simulink model "System23a"  (R2023a)
settings: Solver=ode23t  StartTime=0.0  StopTime=100  MaxStep=0.005  RelTol=1e-3
settings Model: Creator=andriyanov_ilya  LastModifiedBy=Ilya_Andriyanov

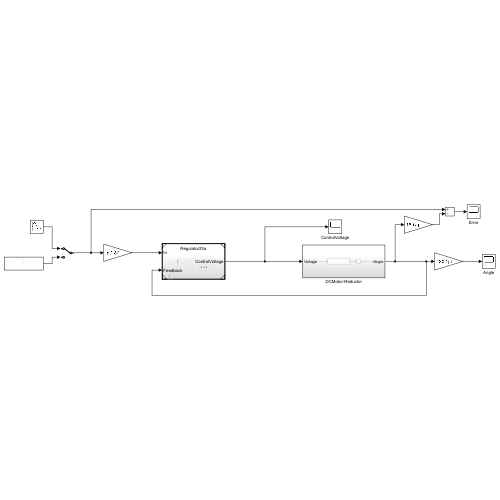
[thumbnail: Simulink's stored preview of the top-level diagram]
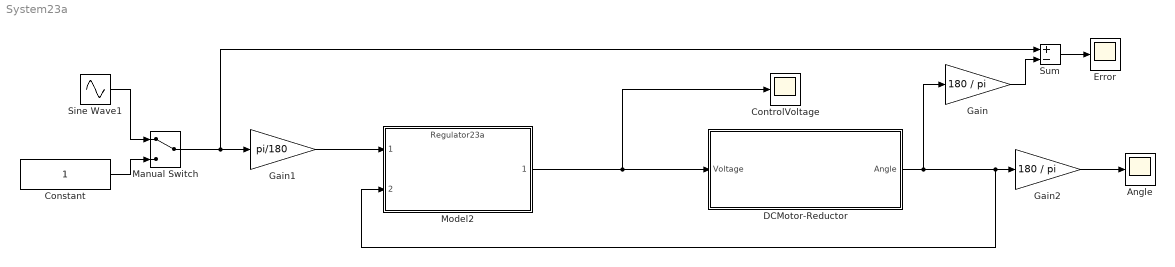
== system System23a ==
  Angle : Scope
  Constant : Constant
  ControlVoltage : Scope
  DCMotor-Reductor : Subsystem
  Error : Scope
  Gain : Gain  Gain=180 / pi
  Gain1 : Gain  Gain=pi/180
  Gain2 : Gain  Gain=180 / pi
  Manual Switch : ManualSwitch
  Model2 : ModelReference  ModelNameDialog=Regulator23a.slx  SimulationMode=Normal  ModelReferenceVersion=1.0
  Sine Wave1 : Sin  Amplitude=140  Frequency=0.63  SampleTime=0
  Sum : Sum  Inputs=+-
  wires:
  DCMotor-Reductor/1(Angle) -> Gain/1, Model2/2, Gain2/1
  Gain/1 -> Sum/2
  Sum/1 -> Error/1
  Constant/1 -> Manual Switch/2
  Sine Wave1/1 -> Manual Switch/1
  Manual Switch/1 -> Sum/1, Gain1/1
  Gain1/1 -> Model2/1
  Model2/1 -> ControlVoltage/1, DCMotor-Reductor/1(Voltage)
  Gain2/1 -> Angle/1

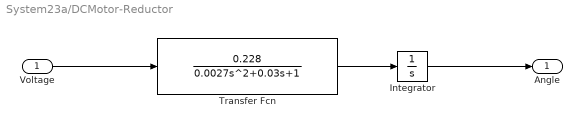
== system System23a/DCMotor-Reductor ==
  Voltage : Inport
  Integrator : Integrator
  Transfer Fcn : TransferFcn  Numerator=[0.228]  Denominator=[0.0027 0.03 1]
  Angle : Outport
  wires:
  Voltage/1 -> Transfer Fcn/1
  Transfer Fcn/1 -> Integrator/1
  Integrator/1 -> Angle/1
